simulink model "Aufgabe4"  (R2015b)
settings: Solver=VariableStepAuto  StartTime=0.0  StopTime=0.005  RelTol=1e-3
InitFcn:
  | Aufgabe4_calc
values from neighbouring files (symbols this model uses):
  duty_cycle = 0.2    [Aufgabe4_calc.m]
  R1 = 1    [Aufgabe4_calc.m]
  R2 = 10E+3    (= 10000)    [Aufgabe4_calc.m]
  R3 = 0.1    [Aufgabe4_calc.m]
  Twidth = 1/f    (= 1e-05)    [Aufgabe4_calc.m]
libraries: fl_lib x11, nesl_utility x5, simulink x2, simulink_extras x1, elec_lib x1
settings Model: Creator=lukaskiechle  LastModifiedBy=lukaskiechle
settings DebuggingCC: MaxConsecutiveZCsMsg=none

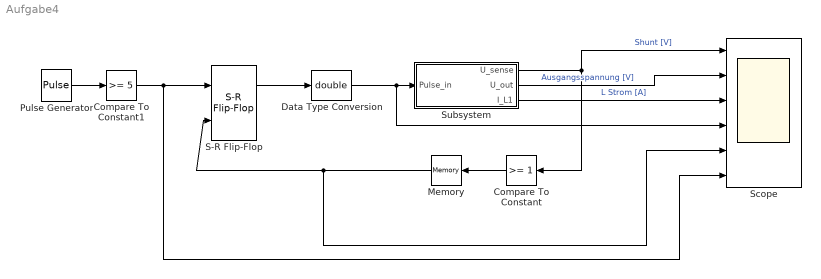
== system Aufgabe4 ==
  Compare To Constant : simulink/Logic and Bit Operations/Compare To Constant  relop=>=  const=1  OutDataTypeStr=boolean  ZeroCross=off
  Compare To Constant1 : simulink/Logic and Bit Operations/Compare To Constant  relop=>=  const=5  OutDataTypeStr=boolean
  Data Type Conversion : DataTypeConversion  OutDataTypeStr=double
  Memory : Memory
  Pulse Generator : DiscretePulseGenerator  PulseType=Time based  Amplitude=10  Period=Twidth  PulseWidth=duty_cycle *100  PhaseDelay=Twidth
  S-R Flip-Flop : simulink_extras/Flip Flops/S-R Flip-Flop  initial_condition=0
  Scope : Scope  NumInputPorts=6
  Subsystem : Subsystem
  wires:
  Subsystem/1(U_sense) -> Compare To Constant/1, Scope/1  "Shunt [V]"
  Subsystem/3(I_L1) -> Scope/3  "L Strom [A]"
  Subsystem/2(U_out) -> Scope/2  "Ausgangsspannung [V]"
  Compare To Constant/1 -> Memory/1
  Memory/1 -> Scope/5, S-R Flip-Flop/2
  Pulse Generator/1 -> Compare To Constant1/1
  Compare To Constant1/1 -> Scope/6, S-R Flip-Flop/1
  S-R Flip-Flop/1 -> Data Type Conversion/1
  Data Type Conversion/1 -> Scope/4, Subsystem/1(Pulse_in)

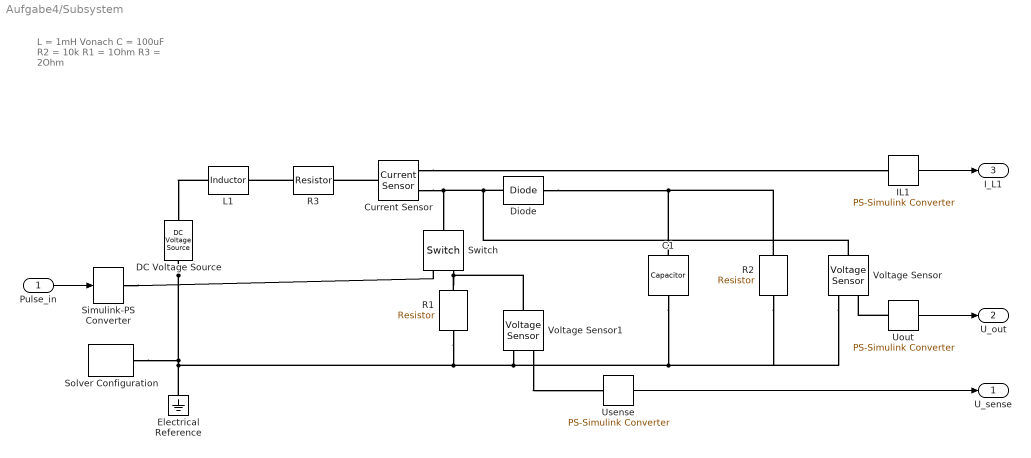
== system Aufgabe4/Subsystem ==
  note: L = 1mH Vonach
      | C = 100uF
      | R2 = 10k
      | R1 = 1Ohm
      | R3 = 2Ohm
  Pulse_in : Inport
  C1 : fl_lib/Electrical/Electrical Elements/Capacitor  c=C1 F  r=1e-6 Ohm  g=0 1/Ohm  i_specify=off  i_priority=None  i=0 A  v_specify=off  v_priority=None  v=0 V  vc_specify=off  vc_priority=None  vc=0 V
  Current Sensor : fl_lib/Electrical/Electrical Sensors/Current Sensor
  DC Voltage Source : fl_lib/Electrical/Electrical Sources/DC Voltage Source  v0=Uin V
  Diode : elec_lib/Semiconductor Devices/Diode  ModelType=2  Vf=0.6 V  Ron=0.1 Ohm  Goff=1e-8 S  Rz=0.1 Ohm  Vz=160 V  C_PWL=5 pF  prmExp=1  I12=[ 0.0137 0.545 ] A  V12=[ 0.6 0.7 ] V  I1=0.0137 A  V1=0.6 V  RS=0.01 Ohm  IS=1e-12 A  Tmeas=25 C  ec=1  BV=Inf V  C_param=1  CJ0=5 pF  VJ=1 V  Mgrad=0.5  Vvec=[ 0.1 10 100 ] V  Cvec=[ 3.5 1 0.4 ] pF  FC=0.5  Q_param=1  Irrm=-7.15 A  iF=4 A  didt=-750 A/us  trr=115 ns  TT=50 ns  tau=100 ns  T_param=1  IS_T2=1.25e-7 A  I1_T2=0.245 A  V1_T2=0.5 V  Tmeas2=125 C  EG_param=1  EG=1.11 eV  XTI_param=1  XTI=3  dBVdT=0 V/K  Tdevice=25 C  Rth=[ 0 10 ] K/W  thermal_mass_parameterization=1  thermal_mass=[ 0 1 ] J/K  thermal_time_constant=[ 0 10 ] s  thermal_mass_initial_temperatures=[ 25 25 ] C
  Electrical Reference : fl_lib/Electrical/Electrical Elements/Electrical Reference
  IL1 : nesl_utility/PS-Simulink Converter  PhysicalDomain=network_engine_domain  SubClassName=ps_output  LeftPortType=input  RightPortType=output  PseudoPeriodic=off  Frequencies=[]  Unit=A  AffineConversion=off
  L1 : fl_lib/Electrical/Electrical Elements/Inductor  l=L1 H  r=0 Ohm  g=1e-9 1/Ohm  i_specify=off  i_priority=None  i=0 A  v_specify=off  v_priority=None  v=0 V  i_L_specify=off  i_L_priority=None  i_L=0 A
  R1 : fl_lib/Electrical/Electrical Elements/Resistor  R=R1 Ohm  i_specify=off  i_priority=None  i=0 A  v_specify=off  v_priority=None  v=0 V
  R2 : fl_lib/Electrical/Electrical Elements/Resistor  R=R2 Ohm  i_specify=off  i_priority=None  i=0 A  v_specify=off  v_priority=None  v=0 V
  R3 : fl_lib/Electrical/Electrical Elements/Resistor  R=R3 Ohm  i_specify=off  i_priority=None  i=0 A  v_specify=off  v_priority=None  v=0 V
  Simulink-PS Converter : nesl_utility/Simulink-PS Converter  PhysicalDomain=network_engine_domain  SubClassName=ps_input  LeftPortType=input  RightPortType=output  PseudoPeriodic=off  Frequencies=[]  NoiseDistribution=none  NoiseParameters=[]  Unit=1  AffineConversion=off  InputFiltering=off  SimscapeFilterOrder=1  InputFilterTimeConstant=0.001  UdotUserProvided=1
  Solver Configuration : nesl_utility/Solver Configuration  PhysicalDomain=network_engine_domain  SubClassName=solver  LeftPortType=input  RightPortType=generic  Accelerate=off  Tones=[]  Harmonics=[]  SimulateNoise=off  Profile=off  UseLocalSampling=off  EnableSwitchedLinearOptims=on  FrequencyDomain=off  UseCCode=off  RelTol=0.001  AbsTol=1e-06  MinStep=1e-09  ToWorkspace=off  RevertToSquareIcSolve=off  NumHomotopyIterations=100  PhasorMode=off  PhasorModeNumHarmonics=1  DoDC=on  ResidualTolerance=1e-09  UseLocalSolver=off  LocalSolverChoice=NE_BACKWARD_EULER_ADVANCER  LocalSolverSampleTime=0.001  DoFixedCost=off  MaxNonlinIter=3  MaxModeIter=2  LinearAlgebra=Sparse  DelaysMemoryBudget=1024  AutomaticFiltering=on  FilteringTimeConstant=0.001
  Switch : fl_lib/Electrical/Electrical Elements/Switch  R_closed=0.01 Ohm  G_open=1e-8 1/Ohm  Threshold=0.5  i_specify=off  i_priority=None  i=0 A  v_specify=off  v_priority=None  v=0 V
  Uout : nesl_utility/PS-Simulink Converter  PhysicalDomain=network_engine_domain  SubClassName=ps_output  LeftPortType=input  RightPortType=output  PseudoPeriodic=off  Frequencies=[]  Unit=V  AffineConversion=off
  Usense : nesl_utility/PS-Simulink Converter  PhysicalDomain=network_engine_domain  SubClassName=ps_output  LeftPortType=input  RightPortType=output  PseudoPeriodic=off  Frequencies=[]  Unit=V  AffineConversion=off
  Voltage Sensor : fl_lib/Electrical/Electrical Sensors/Voltage Sensor
  Voltage Sensor1 : fl_lib/Electrical/Electrical Sensors/Voltage Sensor
  U_sense : Outport
  U_out : Outport  Port=2
  I_L1 : Outport  Port=3
  wires:
  Usense/1 -> U_sense/1
  Uout/1 -> U_out/1
  IL1/1 -> I_L1/1
  Pulse_in/1 -> Simulink-PS Converter/1
  connections:
  Diode/LConn1 -- Current Sensor/RConn2 -- Switch/LConn1 -- Voltage Sensor/LConn1
  DC Voltage Source/RConn1 -- Solver Configuration/RConn1 -- R1/RConn1 -- R2/RConn1 -- Voltage Sensor/RConn2 -- C1/RConn1 -- Voltage Sensor1/RConn2 -- Electrical Reference/LConn1
  C1/LConn1 -- R2/LConn1 -- Diode/RConn1
  Voltage Sensor1/LConn1 -- Switch/RConn2 -- R1/LConn1
  Current Sensor/RConn1 -- IL1/LConn1
  R3/LConn1 -- L1/RConn1
  Current Sensor/LConn1 -- R3/RConn1
  Voltage Sensor1/RConn1 -- Usense/LConn1
  Uout/LConn1 -- Voltage Sensor/RConn1
  L1/LConn1 -- DC Voltage Source/LConn1
  Simulink-PS Converter/RConn1 -- Switch/RConn1
